simulink model "termic_matlab"  (Simulink 7.6)
settings: Solver=ode45  StartTime=0.0  StopTime=7000  RelTol=1e-3
values from neighbouring files (symbols this model uses):
  T = 800    [koef.m]
settings Model: Creator=dpara  LastModifiedBy=Johannes
settings DebuggingCC: StrictBusMsg=Warning

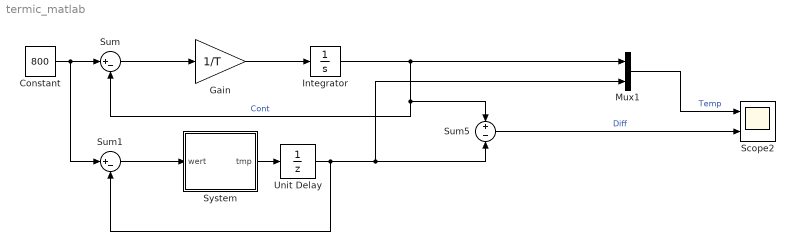
== system termic_matlab ==
  Constant : Constant  Value=800
  Gain : Gain  Gain=1/T
  Integrator : Integrator
  Mux1 : Mux  Inputs=2
  Scope2 : Scope  NumInputPorts=2
      settings: TimeRange=7000  YMin=500~-0.0185  YMax=740~-0.0095  SampleInput=on  SampleTime=1
  Sum : Sum  Inputs=|+-
  Sum1 : Sum  Inputs=|+-
  Sum5 : Sum  Inputs=+-
  System : Stateflow chart  TreatAsAtomicUnit=on  SystemSampleTime=0.1
  Unit Delay : UnitDelay  SampleTime=-1
  wires:
  Constant/1 -> Sum/1, Sum1/1
  Sum/1 -> Gain/1
  Integrator/1 -> Sum/2, Sum5/1, Mux1/1  "Cont"
  Gain/1 -> Integrator/1
  System/1(tmp) -> Unit Delay/1
  Sum5/1 -> Scope2/2  "Diff"
  Mux1/1 -> Scope2/1  "Temp"
  Sum1/1 -> System/1(wert)
  Unit Delay/1 -> Mux1/2, Sum5/2, Sum1/2

== matlab function System ==
  data: wert input double; tmp output double; T parameter double; step parameter double
function tmp = PI(wert,T,step)
    persistent X
    
    if isempty(X)
        X = 0;
    end
    
    X = X + wert/T*step;
    tmp = X;
    
    
%function tmp = PI(wert,K,step) %#eml
    %persistent X
    
    %eml.varsize('X',[1 (7000/0.1+100)]);
    
    %if isempty(X)
    %    X = wert;
    %else
    %    X = [X wert];
    %end;
    
    %res = filter([6.25e-005 6.25e-005],[1 -1],X);
    
    %tmp = res(end);
